simulink library "INP_DMP_Prep"  (R2024b)
settings: Solver=VariableStepAuto  StartTime=0.0  StopTime=10.0  RelTol=1e-3
undefined symbols (not defined in the file): INP_c_TiSample_s, INP_DMP_p_StrkDmpOfsFrLe_mm, INP_DMP_p_StrkDmpScaFrLe_na, INP_p_TiTau_s
libraries: VUT_lib x8
settings Model: Creator=blatak  LastModifiedBy=blatak

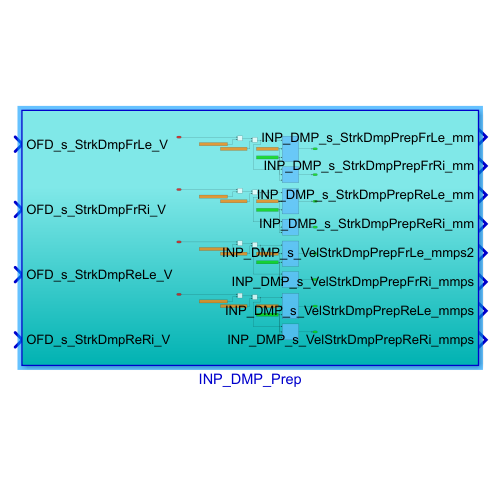
[thumbnail: Simulink's stored preview of the top-level diagram]
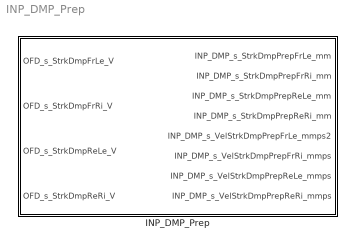
== system INP_DMP_Prep ==
  INP_DMP_Prep : Subsystem

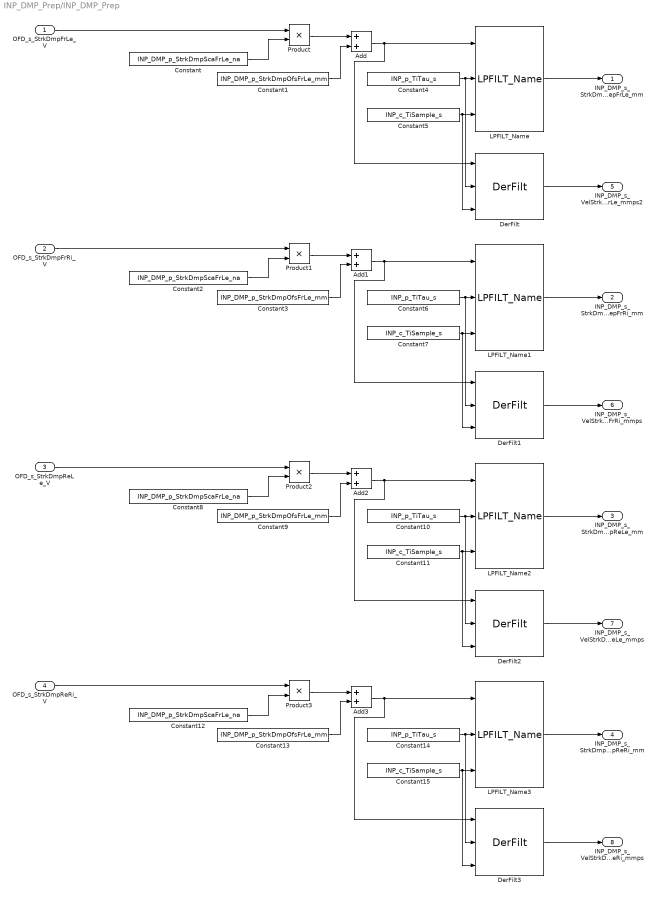
== system INP_DMP_Prep/INP_DMP_Prep ==
  OFD_s_StrkDmpFrLe_V : Inport
  OFD_s_StrkDmpFrRi_V : Inport  Port=2
  OFD_s_StrkDmpReLe_V : Inport  Port=3
  OFD_s_StrkDmpReRi_V : Inport  Port=4
  Add{,1..3} (4 alike) : Sum
  Constant{,2,8,12} (4 alike) : Constant  Description=Scaling coefficient to recalculate the electric quantity to the physical one - longitudinal acceleration  Value=INP_DMP_p_StrkDmpScaFrLe_na
  Constant{1,3,9,13} (4 alike) : Constant  Description=Offset to recalculate the electric quantity to the physical one - longitudinal acceleration  Value=INP_DMP_p_StrkDmpOfsFrLe_mm
  Constant{4,6,10,14} (4 alike) : Constant  Value=INP_p_TiTau_s
  Constant{5,7,11,15} (4 alike) : Constant  Value=INP_c_TiSample_s
  DerFilt{,1..3} (4 alike) : VUT_lib/DerFilt  SystemSampleTime=-1  VariantActivationTime=update diagram  AllowFlexibleInterface=on  Latency=0  AutoFrameSizeCalculation=off
  LPFILT_Name{,1..3} (4 alike) : VUT_lib/LPFILT_Name  SystemSampleTime=-1  VariantActivationTime=update diagram  AllowFlexibleInterface=on  Latency=0  AutoFrameSizeCalculation=off
  Product{,1..3} (4 alike) : Product
  INP_DMP_s_StrkDmpPrepFrLe_mm : Outport
  INP_DMP_s_StrkDmpPrepFrRi_mm : Outport  Port=2
  INP_DMP_s_StrkDmpPrepReLe_mm : Outport  Port=3
  INP_DMP_s_StrkDmpPrepReRi_mm : Outport  Port=4
  INP_DMP_s_VelStrkDmpPrepFrLe_mmps2 : Outport  Port=5
  INP_DMP_s_VelStrkDmpPrepFrRi_mmps : Outport  Port=6
  INP_DMP_s_VelStrkDmpPrepReLe_mmps : Outport  Port=7
  INP_DMP_s_VelStrkDmpPrepReRi_mmps : Outport  Port=8
  wires:
  Constant/1 -> Product/2
  Constant5/1 -> LPFILT_Name/3, DerFilt/3
  Constant1/1 -> Add/2
  Constant4/1 -> LPFILT_Name/2, DerFilt/2
  Add/1 -> LPFILT_Name/1, DerFilt/1
  DerFilt/1 -> INP_DMP_s_VelStrkDmpPrepFrLe_mmps2/1
  Product/1 -> Add/1
  OFD_s_StrkDmpFrLe_V/1 -> Product/1
  LPFILT_Name/1 -> INP_DMP_s_StrkDmpPrepFrLe_mm/1
  Constant7/1 -> LPFILT_Name1/3, DerFilt1/3
  Product1/1 -> Add1/1
  Constant3/1 -> Add1/2
  LPFILT_Name1/1 -> INP_DMP_s_StrkDmpPrepFrRi_mm/1
  DerFilt1/1 -> INP_DMP_s_VelStrkDmpPrepFrRi_mmps/1
  Add1/1 -> LPFILT_Name1/1, DerFilt1/1
  Constant6/1 -> LPFILT_Name1/2, DerFilt1/2
  Constant2/1 -> Product1/2
  OFD_s_StrkDmpFrRi_V/1 -> Product1/1
  Constant11/1 -> LPFILT_Name2/3, DerFilt2/3
  Product2/1 -> Add2/1
  Constant9/1 -> Add2/2
  LPFILT_Name2/1 -> INP_DMP_s_StrkDmpPrepReLe_mm/1
  DerFilt2/1 -> INP_DMP_s_VelStrkDmpPrepReLe_mmps/1
  Add2/1 -> LPFILT_Name2/1, DerFilt2/1
  Constant10/1 -> LPFILT_Name2/2, DerFilt2/2
  Constant8/1 -> Product2/2
  OFD_s_StrkDmpReLe_V/1 -> Product2/1
  Constant15/1 -> LPFILT_Name3/3, DerFilt3/3
  Product3/1 -> Add3/1
  Constant13/1 -> Add3/2
  LPFILT_Name3/1 -> INP_DMP_s_StrkDmpPrepReRi_mm/1
  DerFilt3/1 -> INP_DMP_s_VelStrkDmpPrepReRi_mmps/1
  Add3/1 -> LPFILT_Name3/1, DerFilt3/1
  Constant14/1 -> LPFILT_Name3/2, DerFilt3/2
  Constant12/1 -> Product3/2
  OFD_s_StrkDmpReRi_V/1 -> Product3/1
